simulink model "FrictionCompensation_Development_2024a"  (R2025a)
settings: Solver=FixedStepAuto  StartTime=0.0  StopTime=10  FixedStep=0.002  RelTol=1e-3
settings Model: Creator=Luoyan Peng  LastModifiedBy=Kylo_Ren

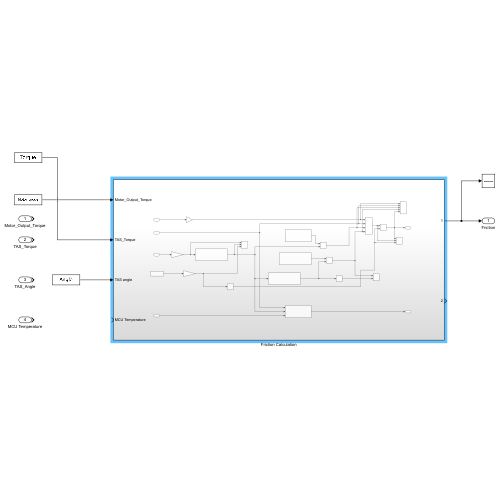
[thumbnail: Simulink's stored preview of the top-level diagram]
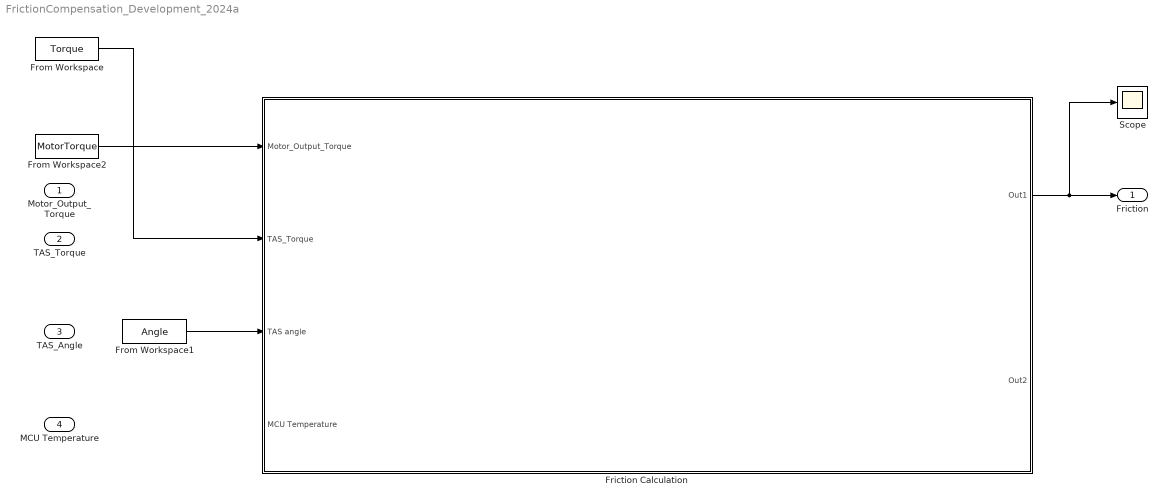
== system FrictionCompensation_Development_2024a ==
  Motor_Output_Torque : Inport
  TAS_Torque : Inport  Port=2
  TAS_Angle : Inport  Port=3
  MCU Temperature : Inport  Port=4
  Friction Calculation : Subsystem
  From Workspace : FromWorkspace  VariableName=Torque
  From Workspace1 : FromWorkspace  VariableName=Angle
  From Workspace2 : FromWorkspace  VariableName=MotorTorque
  Scope : Scope
      settings: ActiveDisplayYMinimum=-1  ActiveDisplayYMaximum=1
  Friction : Outport
  wires:
  Friction Calculation/1(Out1) -> Scope/1, Friction/1
  From Workspace2/1 -> Friction Calculation/1(Motor_Output_Torque)
  From Workspace/1 -> Friction Calculation/2(TAS_Torque)
  From Workspace1/1 -> Friction Calculation/3(TAS angle)

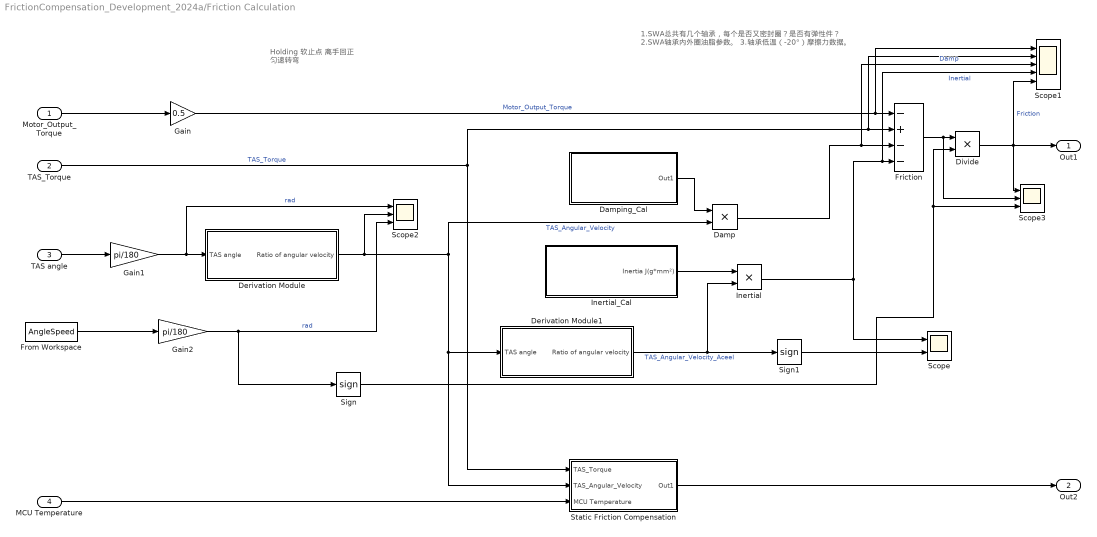
== system FrictionCompensation_Development_2024a/Friction Calculation ==
  note: Holding
      | 软止点
      | 离手回正
      | 匀速转弯
  note: 1.SWA总共有几个轴承，每个是否又密封圈？是否有弹性件？
      | 2.SWA轴承内外圈油脂参数。
      | 3.轴承低温（-20°）摩擦力数据。
  Motor_Output_Torque : Inport
  TAS_Torque : Inport  Port=2
  TAS angle : Inport  Port=3
  MCU Temperature : Inport  Port=4
  Damp : Product  Inputs=**
  Damping_Cal : Subsystem
  Derivation Module : Subsystem
  Derivation Module1 : Subsystem
  Divide : Product  Inputs=**
  Friction : Sum  Inputs=-+--
  From Workspace : FromWorkspace  VariableName=AngleSpeed
  Gain : Gain  Gain=0.5
  Gain1 : Gain  Gain=pi/180
  Gain2 : Gain  Gain=pi/180
  Inertial : Product  Inputs=**
  Inertial_Cal : Subsystem
  Scope : Scope  NumInputPorts=2
      settings: ActiveDisplayYMinimum=-0.00225  ActiveDisplayYMaximum=0.00195
  Scope1 : Scope  NumInputPorts=5
      settings: ActiveDisplayYMinimum=-5.1165282270408161  ActiveDisplayYMaximum=8.5975952729591825  DataLoggingVariableName=ScopeData2
  Scope2 : Scope  NumInputPorts=3
      settings: ActiveDisplayYMinimum=-8.3249079736547  ActiveDisplayYMaximum=11.904669935095301  DataLoggingVariableName=ScopeData3
  Scope3 : Scope  NumInputPorts=3
      settings: ActiveDisplayYMinimum=-1  ActiveDisplayYMaximum=1
  Sign : Signum
  Sign1 : Signum
  Static Friction Compensation : Subsystem
  Out1 : Outport
  Out2 : Outport  Port=2
  wires:
  Damping_Cal/1(Out1) -> Damp/1
  Derivation Module/1(" Ratio of angular velocity") -> Scope2/2, Damp/2, Static Friction Compensation/2(TAS_Angular_Velocity), Derivation Module1/1(TAS angle)  "TAS_Angular_Velocity"
  Inertial/1 -> Scope1/4, Friction/4, Scope/1  "Inertial"
  Friction/1 -> Scope3/2, Divide/1
  TAS angle/1 -> Gain1/1
  Inertial_Cal/1(Inertia J(g*mm²)) -> Inertial/1
  Derivation Module1/1(" Ratio of angular velocity") -> Inertial/2, Sign1/1  "TAS_Angular_Velocity_Aceel"
  Damp/1 -> Scope1/3, Friction/3  "Damp"
  Motor_Output_Torque/1 -> Gain/1
  Static Friction Compensation/1(Out1) -> Out2/1
  MCU Temperature/1 -> Static Friction Compensation/3(MCU Temperature)
  TAS_Torque/1 -> Friction/2, Scope1/2, Static Friction Compensation/1(TAS_Torque)  "TAS_Torque"
  Gain1/1 -> Scope2/1, Derivation Module/1(TAS angle)  "rad"
  From Workspace/1 -> Gain2/1
  Gain2/1 -> Sign/1, Scope2/3  "rad"
  Gain/1 -> Friction/1, Scope1/1  "Motor_Output_Torque"
  Divide/1 -> Scope3/1, Scope1/5, Out1/1  "Friction"
  Sign1/1 -> Scope/2
  Sign/1 -> Scope3/3, Divide/2

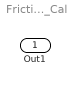
== system FrictionCompensation_Development_2024a/Friction Calculation/Damping_Cal ==
  Out1 : Outport

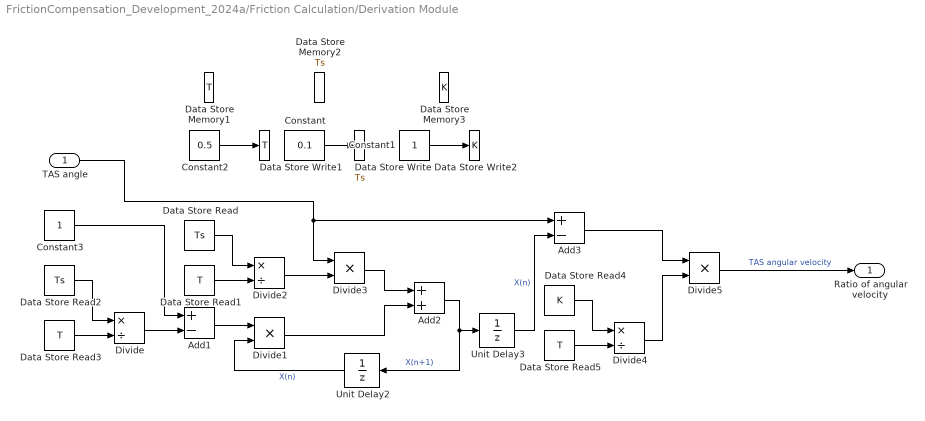
== system FrictionCompensation_Development_2024a/Friction Calculation/Derivation Module ==
  TAS angle : Inport
  Add1 : Sum  Inputs=+-
  Add2 : Sum
  Add3 : Sum  Inputs=+-
  Constant : Constant  Value=0.1
  Constant1 : Constant
  Constant2 : Constant  Value=0.5
  Constant3 : Constant
  Data Store Read : DataStoreRead  DataStoreName=Ts  IndexOptions=Index vector (dialog)  Indices=1  OutputSizes=1
  Data Store Read1 : DataStoreRead  DataStoreName=T  IndexOptions=Index vector (dialog)  Indices=1  OutputSizes=1
  Data Store Read2 : DataStoreRead  DataStoreName=Ts  IndexOptions=Index vector (dialog)  Indices=1  OutputSizes=1
  Data Store Read3 : DataStoreRead  DataStoreName=T  IndexOptions=Index vector (dialog)  Indices=1  OutputSizes=1
  Data Store Read4 : DataStoreRead  DataStoreName=K  IndexOptions=Index vector (dialog)  Indices=1  OutputSizes=1
  Data Store Read5 : DataStoreRead  DataStoreName=T  IndexOptions=Index vector (dialog)  Indices=1  OutputSizes=1
  Data Store Write : DataStoreWrite  DataStoreName=Ts  IndexOptions=Index vector (dialog)  Indices=1  OutputSizes=1
  Data Store Write1 : DataStoreWrite  DataStoreName=T  IndexOptions=Index vector (dialog)  Indices=1  OutputSizes=1
  Data Store Write2 : DataStoreWrite  DataStoreName=K  IndexOptions=Index vector (dialog)  Indices=1  OutputSizes=1
  Data Store Memory1 : DataStoreMemory  DataStoreName=T  ReadBeforeWriteMsg=warning  WriteAfterWriteMsg=warning  WriteAfterReadMsg=warning  ShowAdditionalParam=off
  Data Store Memory2 : DataStoreMemory  DataStoreName=Ts  ReadBeforeWriteMsg=warning  WriteAfterWriteMsg=warning  WriteAfterReadMsg=warning  ShowAdditionalParam=off
  Data Store Memory3 : DataStoreMemory  DataStoreName=K  ReadBeforeWriteMsg=warning  WriteAfterWriteMsg=warning  WriteAfterReadMsg=warning  ShowAdditionalParam=off
  Divide : Product  Inputs=*/
  Divide1 : Product  Inputs=**
  Divide2 : Product  Inputs=*/
  Divide3 : Product  Inputs=**
  Divide4 : Product  Inputs=*/
  Divide5 : Product  Inputs=**
  Unit Delay2 : UnitDelay  SampleTime=-1  HasFrameUpgradeWarning=on
  Unit Delay3 : UnitDelay  SampleTime=-1  HasFrameUpgradeWarning=on
  " Ratio of angular velocity" : Outport
  wires:
  Data Store Read/1 -> Divide2/1
  Divide2/1 -> Divide3/2
  Data Store Read2/1 -> Divide/1
  Constant1/1 -> Data Store Write2/1
  Data Store Read3/1 -> Divide/2
  Constant2/1 -> Data Store Write1/1
  Constant/1 -> Data Store Write/1
  Divide/1 -> Add1/2
  Constant3/1 -> Add1/1
  Unit Delay3/1 -> Add3/2  "X(n)"
  Data Store Read1/1 -> Divide2/2
  Add1/1 -> Divide1/1
  TAS angle/1 -> Add3/1, Divide3/1
  Divide1/1 -> Add2/2
  Unit Delay2/1 -> Divide1/2  "X(n)"
  Data Store Read5/1 -> Divide4/2
  Divide3/1 -> Add2/1
  Add2/1 -> Unit Delay2/1, Unit Delay3/1  "X(n+1)"
  Data Store Read4/1 -> Divide4/1
  Add3/1 -> Divide5/1
  Divide4/1 -> Divide5/2
  Divide5/1 -> " Ratio of angular velocity"/1  "TAS angular velocity"

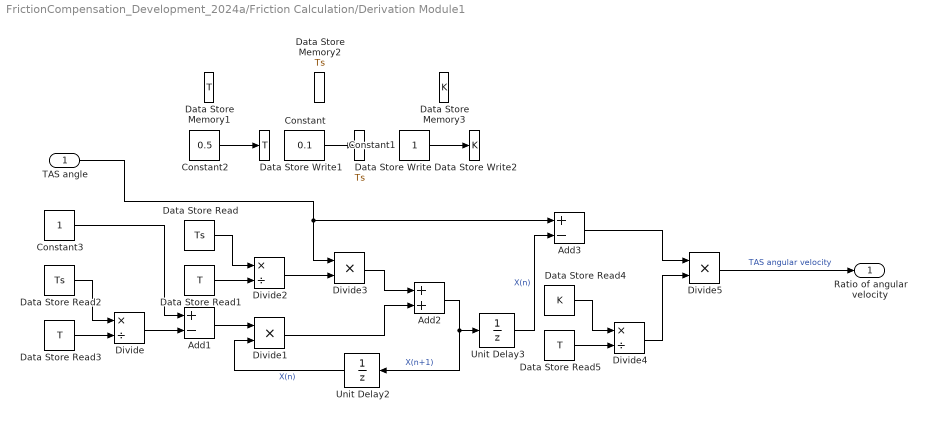
== system FrictionCompensation_Development_2024a/Friction Calculation/Derivation Module1 ==
  TAS angle : Inport
  Add1 : Sum  Inputs=+-
  Add2 : Sum
  Add3 : Sum  Inputs=+-
  Constant : Constant  Value=0.1
  Constant1 : Constant
  Constant2 : Constant  Value=0.5
  Constant3 : Constant
  Data Store Read : DataStoreRead  DataStoreName=Ts  IndexOptions=Index vector (dialog)  Indices=1  OutputSizes=1
  Data Store Read1 : DataStoreRead  DataStoreName=T  IndexOptions=Index vector (dialog)  Indices=1  OutputSizes=1
  Data Store Read2 : DataStoreRead  DataStoreName=Ts  IndexOptions=Index vector (dialog)  Indices=1  OutputSizes=1
  Data Store Read3 : DataStoreRead  DataStoreName=T  IndexOptions=Index vector (dialog)  Indices=1  OutputSizes=1
  Data Store Read4 : DataStoreRead  DataStoreName=K  IndexOptions=Index vector (dialog)  Indices=1  OutputSizes=1
  Data Store Read5 : DataStoreRead  DataStoreName=T  IndexOptions=Index vector (dialog)  Indices=1  OutputSizes=1
  Data Store Write : DataStoreWrite  DataStoreName=Ts  IndexOptions=Index vector (dialog)  Indices=1  OutputSizes=1
  Data Store Write1 : DataStoreWrite  DataStoreName=T  IndexOptions=Index vector (dialog)  Indices=1  OutputSizes=1
  Data Store Write2 : DataStoreWrite  DataStoreName=K  IndexOptions=Index vector (dialog)  Indices=1  OutputSizes=1
  Data Store Memory1 : DataStoreMemory  DataStoreName=T  ReadBeforeWriteMsg=warning  WriteAfterWriteMsg=warning  WriteAfterReadMsg=warning  ShowAdditionalParam=off
  Data Store Memory2 : DataStoreMemory  DataStoreName=Ts  ReadBeforeWriteMsg=warning  WriteAfterWriteMsg=warning  WriteAfterReadMsg=warning  ShowAdditionalParam=off
  Data Store Memory3 : DataStoreMemory  DataStoreName=K  ReadBeforeWriteMsg=warning  WriteAfterWriteMsg=warning  WriteAfterReadMsg=warning  ShowAdditionalParam=off
  Divide : Product  Inputs=*/
  Divide1 : Product  Inputs=**
  Divide2 : Product  Inputs=*/
  Divide3 : Product  Inputs=**
  Divide4 : Product  Inputs=*/
  Divide5 : Product  Inputs=**
  Unit Delay2 : UnitDelay  SampleTime=-1  HasFrameUpgradeWarning=on
  Unit Delay3 : UnitDelay  SampleTime=-1  HasFrameUpgradeWarning=on
  " Ratio of angular velocity" : Outport
  wires:
  Data Store Read/1 -> Divide2/1
  Divide2/1 -> Divide3/2
  Data Store Read2/1 -> Divide/1
  Constant1/1 -> Data Store Write2/1
  Data Store Read3/1 -> Divide/2
  Constant2/1 -> Data Store Write1/1
  Constant/1 -> Data Store Write/1
  Divide/1 -> Add1/2
  Constant3/1 -> Add1/1
  Unit Delay3/1 -> Add3/2  "X(n)"
  Data Store Read1/1 -> Divide2/2
  Add1/1 -> Divide1/1
  TAS angle/1 -> Add3/1, Divide3/1
  Divide1/1 -> Add2/2
  Unit Delay2/1 -> Divide1/2  "X(n)"
  Data Store Read5/1 -> Divide4/2
  Divide3/1 -> Add2/1
  Add2/1 -> Unit Delay2/1, Unit Delay3/1  "X(n+1)"
  Data Store Read4/1 -> Divide4/1
  Add3/1 -> Divide5/1
  Divide4/1 -> Divide5/2
  Divide5/1 -> " Ratio of angular velocity"/1  "TAS angular velocity"

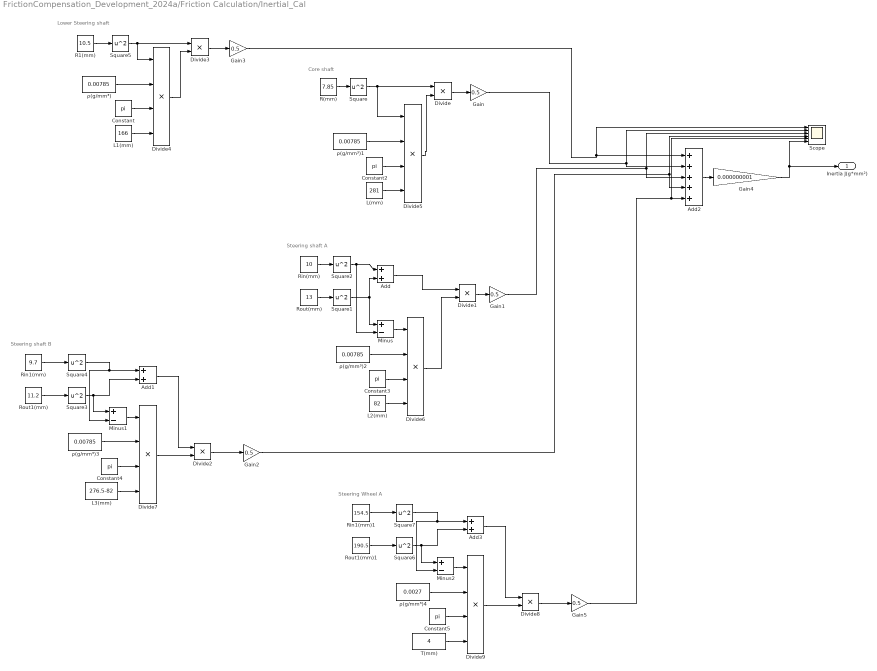
== system FrictionCompensation_Development_2024a/Friction Calculation/Inertial_Cal ==
  note: Steering shaft A
  note: Core shaft
  note: Steering shaft B
  note: Lower Steering shaft
  note: Steering Wheel A
  Add : Sum
  Add1 : Sum
  Add2 : Sum  Inputs=+++++
  Add3 : Sum
  Constant{,2..5} (5 alike) : Constant  Value=pi
  Divide{,1..3,8} (5 alike) : Product  Inputs=**
  Divide{4..7,9} (5 alike) : Product  Inputs=****
  Gain{,1..3,5} (5 alike) : Gain  Gain=0.5
  Gain4 : Gain  Gain=0.000000001
  L(mm) : Constant  Value=281
  L1(mm) : Constant  Value=166
  L2(mm) : Constant  Value=82
  L3(mm) : Constant  Value=276.5-82
  Minus : Sum  Inputs=+-
  Minus1 : Sum  Inputs=+-
  Minus2 : Sum  Inputs=+-
  R(mm) : Constant  Value=7.85
  R1(mm) : Constant  Value=10.5
  Rin(mm) : Constant  Value=10
  Rin1(mm) : Constant  Value=9.7
  Rin1(mm)1 : Constant  Value=154.5
  Rout(mm) : Constant  Value=13
  Rout1(mm) : Constant  Value=11.2
  Rout1(mm)1 : Constant  Value=190.5
  Scope : Scope  NumInputPorts=6
      settings: ActiveDisplayYMinimum=-1.58447968183E+6  ActiveDisplayYMaximum=1.426031726398E+7  DataLoggingVariableName=ScopeData4
  Square{,1..7} (8 alike) : Math  Operator=square
  T(mm) : Constant  Value=4
  ρ(g/mm³){,1..3} (4 alike) : Constant  Value=0.00785
  ρ(g/mm³)4 : Constant  Value=0.0027
  Inertia J(g*mm²) : Outport
  wires:
  R(mm)/1 -> Square/1
  Square/1 -> Divide5/1, Divide/1
  Divide/1 -> Gain/1
  Divide1/1 -> Gain1/1
  Rout(mm)/1 -> Square1/1
  Square1/1 -> Minus/1, Add/2
  Rin(mm)/1 -> Square2/1
  Square2/1 -> Add/1, Minus/2
  Add/1 -> Divide1/1
  Rout1(mm)/1 -> Square3/1
  Divide2/1 -> Gain2/1
  Rin1(mm)/1 -> Square4/1
  Add1/1 -> Divide2/1
  L1(mm)/1 -> Divide4/4
  Divide3/1 -> Gain3/1
  R1(mm)/1 -> Square5/1
  Square5/1 -> Divide4/1, Divide3/1
  Gain/1 -> Scope/2, Add2/2
  Gain3/1 -> Scope/1, Add2/1
  Gain1/1 -> Scope/3, Add2/3
  Gain2/1 -> Scope/4, Add2/4
  Add2/1 -> Gain4/1
  ρ(g/mm³)/1 -> Divide4/2
  Constant/1 -> Divide4/3
  Divide4/1 -> Divide3/2
  L(mm)/1 -> Divide5/4
  ρ(g/mm³)1/1 -> Divide5/2
  Constant2/1 -> Divide5/3
  Divide5/1 -> Divide/2
  ρ(g/mm³)2/1 -> Divide6/2
  Constant3/1 -> Divide6/3
  L2(mm)/1 -> Divide6/4
  Minus/1 -> Divide6/1
  Divide6/1 -> Divide1/2
  Constant4/1 -> Divide7/3
  Square4/1 -> Minus1/2, Add1/1
  Divide7/1 -> Divide2/2
  Minus1/1 -> Divide7/1
  Square3/1 -> Minus1/1, Add1/2
  ρ(g/mm³)3/1 -> Divide7/2
  L3(mm)/1 -> Divide7/4
  Gain4/1 -> Scope/6, Inertia J(g*mm²)/1
  Square7/1 -> Minus2/2, Add3/1
  Add3/1 -> Divide8/1
  Minus2/1 -> Divide9/1
  Constant5/1 -> Divide9/3
  ρ(g/mm³)4/1 -> Divide9/2
  Square6/1 -> Minus2/1, Add3/2
  Divide9/1 -> Divide8/2
  Divide8/1 -> Gain5/1
  T(mm)/1 -> Divide9/4
  Rout1(mm)1/1 -> Square6/1
  Rin1(mm)1/1 -> Square7/1
  Gain5/1 -> Scope/5, Add2/5

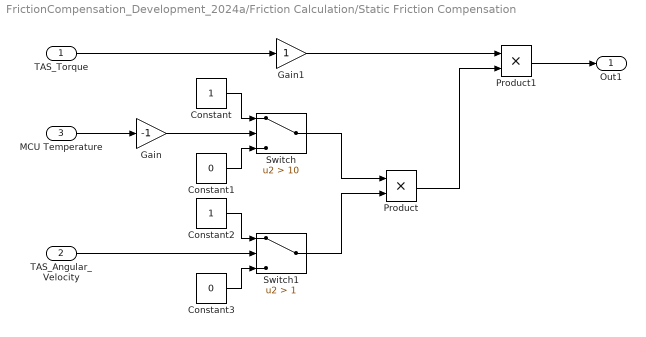
== system FrictionCompensation_Development_2024a/Friction Calculation/Static Friction Compensation ==
  TAS_Torque : Inport
  TAS_Angular_Velocity : Inport  Port=2
  MCU Temperature : Inport  Port=3
  Constant : Constant
  Constant1 : Constant  Value=0
  Constant2 : Constant
  Constant3 : Constant  Value=0
  Gain : Gain  Gain=-1
  Gain1 : Gain
  Product : Product
  Product1 : Product
  Switch : Switch  Criteria=u2 > Threshold  Threshold=10  SaturateOnIntegerOverflow=off  InputSameDT=off
  Switch1 : Switch  Criteria=u2 > Threshold  Threshold=1  SaturateOnIntegerOverflow=off  InputSameDT=off
  Out1 : Outport
  wires:
  MCU Temperature/1 -> Gain/1
  Gain/1 -> Switch/2
  Constant/1 -> Switch/1
  Constant1/1 -> Switch/3
  TAS_Angular_Velocity/1 -> Switch1/2
  Constant2/1 -> Switch1/1
  Constant3/1 -> Switch1/3
  Switch1/1 -> Product/2
  Switch/1 -> Product/1
  Product/1 -> Product1/2
  TAS_Torque/1 -> Gain1/1
  Gain1/1 -> Product1/1
  Product1/1 -> Out1/1
